simulink model "diagrama_de_bloques"  (R2017b)
settings: Solver=FixedStepDiscrete  StartTime=0.0  StopTime=erle.T_simulacion  FixedStep=erle.Tm  RelTol=1e-3
undefined symbols (not defined in the file or in its folder): erle
settings Model: Creator=javi  LastModifiedBy=javi
settings DataIOCC: SaveFormat=Array

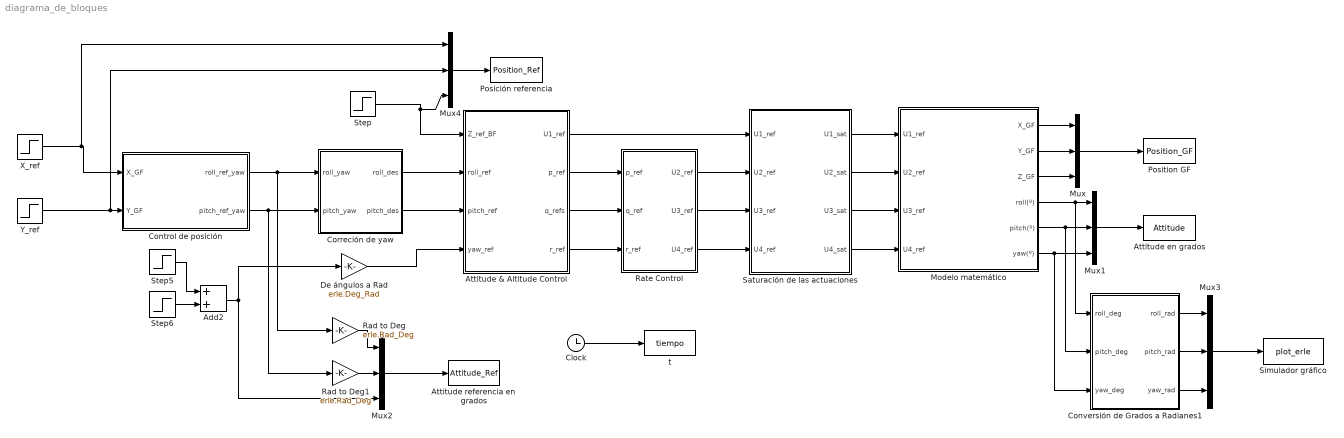
== system diagrama_de_bloques ==
  Add2 : Sum
  Attitude & Altitude Control : Subsystem
  Attitude en grados : ToWorkspace  VariableName=Attitude  SampleTime=erle.Tm
  Attitude referencia en grados : ToWorkspace  VariableName=Attitude_Ref  SampleTime=erle.Tm
  Clock : Clock
  Control de posición : Subsystem
  Conversión de Grados a Radianes1 : Subsystem
  Correción de yaw : Subsystem
  De ángulos a Rad : Gain  Gain=erle.Deg_Rad
  Modelo matemático : Subsystem
  Mux{,1..4} (5 alike) : Mux  Inputs=3
  Posición referencia : ToWorkspace  VariableName=Position_Ref  SampleTime=erle.Tm
  Position GF : ToWorkspace  VariableName=Position_GF  SampleTime=erle.Tm
  Rad to Deg : Gain  Gain=erle.Rad_Deg
  Rad to Deg1 : Gain  Gain=erle.Rad_Deg
  Rate Control : Subsystem
  Saturación de las actuaciones : Subsystem
  Simulador gráfico : MATLABFcn  MATLABFcn=plot_erle  OutputDimensions=0
  Step : Step  SampleTime=erle.Tm
  Step5 : Step  Time=6  After=0  SampleTime=erle.Tm
  Step6 : Step  Time=8  After=0  SampleTime=erle.Tm
  X_ref : Step  Time=erle.X_t  After=erle.X_des  SampleTime=erle.Tm
  Y_ref : Step  Time=erle.Y_t  After=erle.Y_des  SampleTime=erle.Tm
  "t " : ToWorkspace  VariableName=tiempo  SampleTime=erle.Tm
  wires:
  Attitude & Altitude Control/2(p_ref) -> Rate Control/1(p_ref)
  Attitude & Altitude Control/3(q_refs) -> Rate Control/2(q_ref)
  Attitude & Altitude Control/4(r_ref) -> Rate Control/3(r_ref)
  Attitude & Altitude Control/1(U1_ref) -> Saturación de las actuaciones/1(U1_ref)
  Rate Control/1(U2_ref) -> Saturación de las actuaciones/2(U2_ref)
  Rate Control/2(U3_ref) -> Saturación de las actuaciones/3(U3_ref)
  Rate Control/3(U4_ref) -> Saturación de las actuaciones/4(U4_ref)
  Saturación de las actuaciones/1(U1_sat) -> Modelo matemático/1(U1_ref)
  Saturación de las actuaciones/2(U2_sat) -> Modelo matemático/2(U2_ref)
  Saturación de las actuaciones/3(U3_sat) -> Modelo matemático/3(U3_ref)
  Saturación de las actuaciones/4(U4_sat) -> Modelo matemático/4(U4_ref)
  Modelo matemático/1(X_GF) -> Mux/1
  Modelo matemático/2(Y_GF) -> Mux/2
  Modelo matemático/3(Z_GF) -> Mux/3
  Mux/1 -> Position GF/1
  Modelo matemático/4(roll(º)) -> Conversión de Grados a Radianes1/1(roll_deg), Mux1/1
  Modelo matemático/6(yaw(º)) -> Conversión de Grados a Radianes1/3(yaw_deg), Mux1/3
  Mux1/1 -> Attitude en grados/1
  Modelo matemático/5(pitch(º)) -> Conversión de Grados a Radianes1/2(pitch_deg), Mux1/2
  Step/1 -> Mux4/3, Attitude & Altitude Control/1(Z_ref_BF)
  Correción de yaw/1(roll_des) -> Attitude & Altitude Control/2(roll_ref)
  Correción de yaw/2(pitch_des) -> Attitude & Altitude Control/3(pitch_ref)
  De ángulos a Rad/1 -> Attitude & Altitude Control/4(yaw_ref)
  Step6/1 -> Add2/2
  Step5/1 -> Add2/1
  Clock/1 -> "t "/1
  Add2/1 -> De ángulos a Rad/1, Mux2/3
  Mux2/1 -> Attitude referencia en grados/1
  Conversión de Grados a Radianes1/1(roll_rad) -> Mux3/1
  Conversión de Grados a Radianes1/2(pitch_rad) -> Mux3/2
  Conversión de Grados a Radianes1/3(yaw_rad) -> Mux3/3
  Mux3/1 -> Simulador gráfico/1
  Control de posición/1(roll_ref_yaw) -> Rad to Deg/1, Correción de yaw/1(roll_yaw)
  Control de posición/2(pitch_ref_yaw) -> Rad to Deg1/1, Correción de yaw/2(pitch_yaw)
  Rad to Deg1/1 -> Mux2/2
  Rad to Deg/1 -> Mux2/1
  X_ref/1 -> Mux4/1, Control de posición/1(X_GF)
  Mux4/1 -> Posición referencia/1
  Y_ref/1 -> Mux4/2, Control de posición/2(Y_GF)

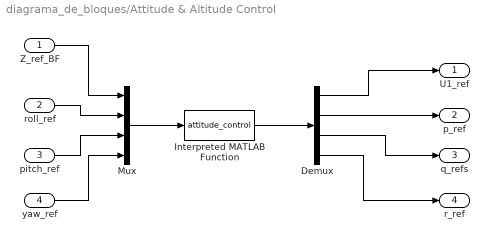
== system diagrama_de_bloques/Attitude & Altitude Control ==
  Z_ref_BF : Inport
  roll_ref : Inport  Port=2
  pitch_ref : Inport  Port=3
  yaw_ref : Inport  Port=4
  Demux : Demux
  Interpreted MATLAB Function : MATLABFcn  MATLABFcn=attitude_control
  Mux : Mux
  U1_ref : Outport
  p_ref : Outport  Port=2
  q_refs : Outport  Port=3
  r_ref : Outport  Port=4
  wires:
  Demux/4 -> r_ref/1
  yaw_ref/1 -> Mux/4
  Demux/1 -> U1_ref/1
  Mux/1 -> Interpreted MATLAB Function/1
  Demux/3 -> q_refs/1
  Interpreted MATLAB Function/1 -> Demux/1
  pitch_ref/1 -> Mux/3
  Demux/2 -> p_ref/1
  Z_ref_BF/1 -> Mux/1
  roll_ref/1 -> Mux/2

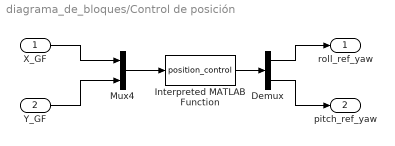
== system diagrama_de_bloques/Control de posición ==
  X_GF : Inport
  Y_GF : Inport  Port=2
  Demux : Demux  Outputs=2
  Interpreted MATLAB Function : MATLABFcn  MATLABFcn=position_control
  Mux4 : Mux  Inputs=2
  roll_ref_yaw : Outport
  pitch_ref_yaw : Outport  Port=2
  wires:
  Y_GF/1 -> Mux4/2
  Interpreted MATLAB Function/1 -> Demux/1
  Demux/2 -> pitch_ref_yaw/1
  Demux/1 -> roll_ref_yaw/1
  Mux4/1 -> Interpreted MATLAB Function/1
  X_GF/1 -> Mux4/1

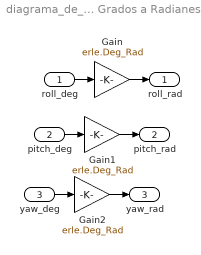
== system diagrama_de_bloques/Conversión de Grados a Radianes1 ==
  roll_deg : Inport
  pitch_deg : Inport  Port=2
  yaw_deg : Inport  Port=3
  Gain : Gain  Gain=erle.Deg_Rad
  Gain1 : Gain  Gain=erle.Deg_Rad
  Gain2 : Gain  Gain=erle.Deg_Rad
  roll_rad : Outport
  pitch_rad : Outport  Port=2
  yaw_rad : Outport  Port=3
  wires:
  Gain2/1 -> yaw_rad/1
  Gain/1 -> roll_rad/1
  roll_deg/1 -> Gain/1
  yaw_deg/1 -> Gain2/1
  pitch_deg/1 -> Gain1/1
  Gain1/1 -> pitch_rad/1

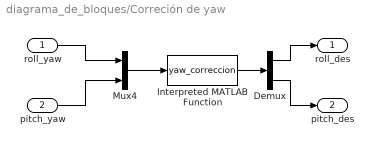
== system diagrama_de_bloques/Correción de yaw ==
  roll_yaw : Inport
  pitch_yaw : Inport  Port=2
  Demux : Demux  Outputs=2
  Interpreted MATLAB Function : MATLABFcn  MATLABFcn=yaw_correccion
  Mux4 : Mux  Inputs=2
  roll_des : Outport
  pitch_des : Outport  Port=2
  wires:
  Interpreted MATLAB Function/1 -> Demux/1
  Demux/2 -> pitch_des/1
  Mux4/1 -> Interpreted MATLAB Function/1
  roll_yaw/1 -> Mux4/1
  Demux/1 -> roll_des/1
  pitch_yaw/1 -> Mux4/2

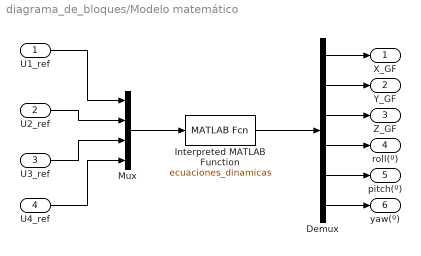
== system diagrama_de_bloques/Modelo matemático ==
  U1_ref : Inport
  U2_ref : Inport  Port=2
  U3_ref : Inport  Port=3
  U4_ref : Inport  Port=4
  Demux : Demux  Outputs=6
  Interpreted MATLAB Function : MATLABFcn  MATLABFcn=ecuaciones_dinamicas
  Mux : Mux
  X_GF : Outport
  Y_GF : Outport  Port=2
  Z_GF : Outport  Port=3
  roll(º) : Outport  Port=4
  pitch(º) : Outport  Port=5
  yaw(º) : Outport  Port=6
  wires:
  U3_ref/1 -> Mux/3
  Mux/1 -> Interpreted MATLAB Function/1
  U2_ref/1 -> Mux/2
  U4_ref/1 -> Mux/4
  U1_ref/1 -> Mux/1
  Interpreted MATLAB Function/1 -> Demux/1
  Demux/1 -> X_GF/1
  Demux/2 -> Y_GF/1
  Demux/3 -> Z_GF/1
  Demux/4 -> roll(º)/1
  Demux/5 -> pitch(º)/1
  Demux/6 -> yaw(º)/1

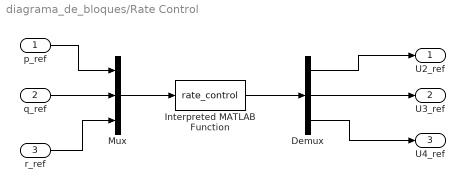
== system diagrama_de_bloques/Rate Control ==
  p_ref : Inport
  q_ref : Inport  Port=2
  r_ref : Inport  Port=3
  Demux : Demux  Outputs=3
  Interpreted MATLAB Function : MATLABFcn  MATLABFcn=rate_control
  Mux : Mux  Inputs=3
  U2_ref : Outport
  U3_ref : Outport  Port=2
  U4_ref : Outport  Port=3
  wires:
  Demux/3 -> U4_ref/1
  Interpreted MATLAB Function/1 -> Demux/1
  Demux/1 -> U2_ref/1
  q_ref/1 -> Mux/2
  Demux/2 -> U3_ref/1
  p_ref/1 -> Mux/1
  r_ref/1 -> Mux/3
  Mux/1 -> Interpreted MATLAB Function/1

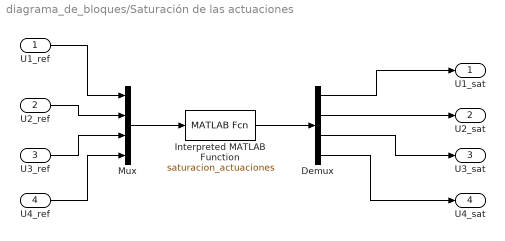
== system diagrama_de_bloques/Saturación de las actuaciones ==
  U1_ref : Inport
  U2_ref : Inport  Port=2
  U3_ref : Inport  Port=3
  U4_ref : Inport  Port=4
  Demux : Demux
  Interpreted MATLAB Function : MATLABFcn  MATLABFcn=saturacion_actuaciones
  Mux : Mux
  U1_sat : Outport
  U2_sat : Outport  Port=2
  U3_sat : Outport  Port=3
  U4_sat : Outport  Port=4
  wires:
  Demux/1 -> U1_sat/1
  Interpreted MATLAB Function/1 -> Demux/1
  Demux/2 -> U2_sat/1
  U3_ref/1 -> Mux/3
  Demux/3 -> U3_sat/1
  U4_ref/1 -> Mux/4
  U2_ref/1 -> Mux/2
  U1_ref/1 -> Mux/1
  Demux/4 -> U4_sat/1
  Mux/1 -> Interpreted MATLAB Function/1
